simulink model "my_second_model"  (R2019b)
settings: Solver=VariableStepAuto  StartTime=0.0  StopTime=10.0  RelTol=1e-3
libraries: simulink x1
settings Model: Creator=Pranshu  LastModifiedBy=Pranshu

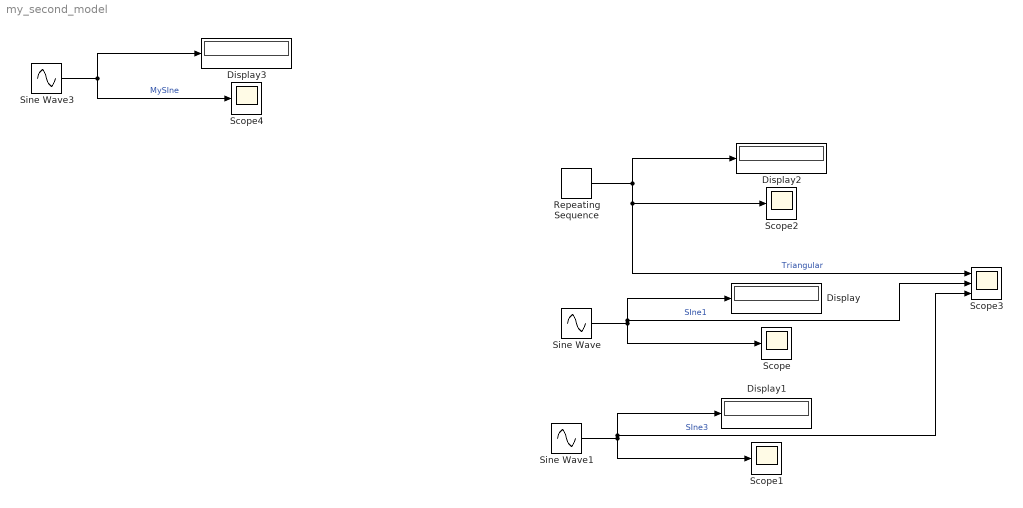
== system my_second_model ==
  Display{,1..3} (4 alike) : Display
  Repeating Sequence : simulink/Sources/Repeating Sequence  rep_seq_t=[0 2]  rep_seq_y=[0 2]
  Scope{,1..2,4} (4 alike) : Scope
  Scope3 : Scope  NumInputPorts=3
  Sine Wave : Sin  Amplitude=3  Frequency=5  SampleTime=0
  Sine Wave1 : Sin  SampleTime=0
  Sine Wave3 : Sin  Amplitude=3  Frequency=5  SampleTime=0
  wires:
  Sine Wave/1 -> Scope3/2, Display/1, Scope/1  "SIne1"
  Sine Wave1/1 -> Scope3/3, Display1/1, Scope1/1  "SIne3"
  Repeating Sequence/1 -> Display2/1, Scope3/1, Scope2/1  "Triangular"
  Sine Wave3/1 -> Display3/1, Scope4/1  "MySIne"
